simulink model "testemplanner_cs"  (R2023a)
settings: Solver=ode5  StartTime=0.0  StopTime=60  FixedStep=1/1000  RelTol=1e-3
PreLoadFcn:
  | mbxruntime.callbacks.PreLoadFcn(bdroot);
PostLoadFcn:
  | mbxruntime.callbacks.PostLoadFcn(bdroot);
InitFcn:
  | mbxruntime.callbacks.InitFcn(bdroot);
StartFcn:
  | mbxruntime.callbacks.StartFcn(bdroot);
StopFcn:
  | mbxruntime.callbacks.StopFcn(bdroot);
model workspace (MAT data in the model file):
  mbox_table : object (value not decoded)
  model_closed = 0
  sim_status = 0
undefined symbols (not defined in the file): aubr, c_factor, cf, cr, DiscIntNeverNeededParam, global_path_x, global_path_y, KD_PID_distance, KD_PID_speed, KI_PID_distance, KI_PID_speed, KP_PID_distance, KP_PID_speed, la, lb, LQR_K1, LQR_K2, LQR_K3, LQR_K4, m, rack_displacement, right_wheel_ground, tablebr, vubr, vx_break_point
libraries: PreScanSimulinkLibrary x14, Solver_SF x1
(part 7 of 8)

== matlab function testemplanner_cs/Audi_A8_Sedan_1/decision&planning module1/EM Planner/Generate Convex Space&Quadratic Programming/path planning with quadratic programming (qp) ==
  data: qp_path_s output; l_min input; qp_path_l output; l_max input; w_cost_l input; w_cost_dl input; w_cost_ddl input; w_cost_dddl input; w_cost_centre input; w_cost_end_l input; w_cost_end_dl input; w_cost_end_ddl input; host_d1 input; host_d2 input; host_w input; plan_start_s input; plan_start_l input; plan_start_dl input; plan_start_ddl input; qp_path_dl output; qp_path_ddl output; delta_dl_max input; delta_ddl_max input
function [qp_path_s,qp_path_l,qp_path_dl,qp_path_ddl] = ...
fcn(l_min,l_max,w_cost_l,w_cost_dl,w_cost_ddl,w_cost_dddl,w_cost_centre,w_cost_end_l,w_cost_end_dl,w_cost_end_ddl,...
    host_d1,host_d2,host_w,...
    plan_start_s,plan_start_l,plan_start_dl,plan_start_ddl,...
    delta_dl_max,delta_ddl_max)
% 路径二次规划
% 0.5*x'Hx + f'*x = min
% subject to A*x <= b
%            Aeq*x = beq
%            lb <= x <= ub;
% 输入：l_min l_max 点的凸空间
%       w_cost_l 参考线代价
%       w_cost_dl ddl dddl 光滑性代价
%       w_cost_centre 凸空间中央代价
%       w_cost_end_l dl dd1 终点的状态代价 (希望path的终点状态为(0,0,0))
%       host_d1,d2 host质心到前后轴的距离
%       host_w host的宽度
%       plan_start_l,dl,ddl 规划起点
% 输出 qp_path_l dl ddl 二次规划输出的曲线
coder.extrinsic("quadprog");
% 待优化的变量的数量
n = 20;

% 输出初始化
qp_path_l = zeros(n,1);
qp_path_dl = zeros(n,1);
qp_path_ddl = zeros(n,1);
qp_path_s = zeros(n,1);

% H_L H_DL H_DDL H_DDDL Aeq beq A b 初始化
H_L = zeros(3*n, 3*n);
H_DL = zeros(3*n, 3*n);
H_DDL = zeros(3*n, 3*n);
H_DDDL = zeros(n-1, 3*n);
H_CENTRE = zeros(3*n, 3*n);
H_L_END = zeros(3*n, 3*n);
H_DL_END = zeros(3*n, 3*n);
H_DDL_END = zeros(3*n, 3*n);
Aeq = zeros(2*n-2, 3*n);
beq = zeros(2*n-2, 1);
A = zeros(8*n, 3*n);
b = zeros(8*n, 1);
% 更新：加入 dl(i+1) - dl(i) ddl(i+1) - ddl(i) 的约束
A_dl_minus = zeros(n - 1,3*n);
b_dl_minus = zeros(n - 1,1);
A_ddl_minus = zeros(n - 1,3*n);
b_ddl_minus = zeros(n - 1,1);
for i = 1:n-1
    row = i;
    col = 3*i - 2;
    A_dl_minus(row,col:col+5) = [0 -1 0 0 1 0];
    b_dl_minus(row) = delta_dl_max;
    A_ddl_minus(row,col:col+5) = [0 0 -1 0 0 1];
    b_ddl_minus(row) = delta_ddl_max;
end
% -max < a*x < max => ax < max && -ax < -(-max)
A_minus = [A_dl_minus;
          -A_dl_minus;
           A_ddl_minus;
          -A_ddl_minus];
b_minus = [b_dl_minus;
           b_dl_minus;
          b_ddl_minus;
          b_ddl_minus]; 

%  期望的终点状态
end_l_desire = 0;
end_dl_desire = 0;
end_ddl_desire = 0;

% Aeq_sub
ds = 3;%纵向间隔
for i = 1:n
    qp_path_s(i) = plan_start_s + (i-1)*ds;
end

Aeq_sub = [1 ds ds^2/3 -1 0 ds^2/6;
           0 1  ds/2   0 -1 ds/2];
% A_sub;
d1 = host_d1;
d2 = host_d2;
w = host_w;
A_sub = [1  d1 0;
         1  d1 0;
         1 -d2 0;
         1 -d2 0;
        -1 -d1 0;
        -1 -d1 0;
        -1  d2 0;
        -1  d2 0];
% 生成Aeq
for i = 1:n-1
    % 计算分块矩阵左上角的行和列
    row = 2*i - 1;
    col = 3*i - 2;
    Aeq(row:row + 1,col:col + 5) = Aeq_sub;
end
% 生成A
for i = 2:n
    row = 8*i - 7;
    col = 3*i - 2;
    A(row:row + 7,col:col + 2) = A_sub;
end

% 视频里用的找(s(i) - d2,s(i) + d1)的方法过于保守，在这里舍弃掉
% 只要找到四个角点所对应的l_min l_max 即可
% 。。。。。。。。。。。。。。
%    [    .   ]<- 
%    [        ]
% 。。。。。。。。。。。。。
front_index = ceil(d1/ds);
back_index = ceil(d2/ds); % ceil向上取整 ceil(3) = 3 ceil(3.1) = 4
% 生成b
for i = 2:n
    % 左前 右前的index = min(i + front_index,60)
    % 左后 右后的index = max(i - back_index,1)
    % l_min l_max 都是60个点
    index1 = min(3*i - 2 + front_index,n);
    index2 = max(3*i - 2 - back_index,1);
    b(8*i - 7:8*i,1) = [l_max(index1) - w/2;
                        l_max(index1) + w/2;
                        l_max(index2) - w/2;
                        l_max(index2) + w/2;
                       -l_min(index1) + w/2;
                       -l_min(index1) - w/2;
                       -l_min(index2) + w/2;
                       -l_min(index2) - w/2;];
end
%生成 lb ub 主要是对规划起点做约束
lb = ones(3*n,1)*-inf;
ub = ones(3*n,1)*inf;
lb(1) = plan_start_l;
lb(2) = plan_start_dl;
lb(3) = plan_start_ddl;
ub(1) = lb(1);
ub(2) = lb(2);
ub(3) = lb(3);
for i = 2:n
    lb(3*i - 1) = - 2; %约束 l'
    ub(3*i - 1) = 2;
    lb(3*i) = -0.1; %约束 l''
    ub(3*i) = 0.1;
end
% 生成H_L,H_DL,H_DDL,H_CENTRE
for i = 1:n
    H_L(3*i - 2,3*i - 2) = 1;
    H_DL(3*i - 1,3*i - 1) = 1;
    H_DDL(3*i, 3*i) = 1;
end
H_CENTRE = H_L;
% 生成H_DDDL;
H_dddl_sub = [0 0 1 0 0 -1];
for i = 1:n-1
    row = i;
    col = 3*i - 2;
    H_DDDL(row,col:col + 5) = H_dddl_sub;
end
% 生成H_L_END H_DL_END H_DDL_END
H_L_END(3*n - 2,3*n - 2) = 1;
H_DL_END(3*n - 1,3*n - 1) = 1;
H_DDL_END(3*n,3*n) = 1;
% 生成二次规划的H 因为ds ！= 1 所以 dddl = delta_ddl/ds;
H = w_cost_l * (H_L'*H_L) + w_cost_dl * (H_DL'*H_DL) + w_cost_ddl * (H_DDL'*H_DDL)...
   +w_cost_dddl * (H_DDDL'*H_DDDL)/ds + w_cost_centre * (H_CENTRE'*H_CENTRE) + w_cost_end_l * (H_L_END'*H_L_END)...
   +w_cost_end_dl * (H_DL_END'* H_DL_END) + w_cost_ddl * (H_DDL_END'*H_DDL_END);
H = 2 * H;
% 生成f
f = zeros(3*n,1);
 centre_line = 0.5 * (l_min + l_max); % 此时centre line 还是60个点
% centre_line = dp_path_l_final;
for i = 1:n
    f(3*i - 2) = -2 * centre_line(3*i - 2);
end
% 避免centreline权重过大影响轨迹平顺性
for i = 1:n
    if abs(f(i)) > 0.3
        f(i) = w_cost_centre * f(i);
    end
end
% 终点要接近end_l dl ddl desire
f(3*n - 2) = f(3*n - 2) -2 * end_l_desire * w_cost_end_l;
f(3*n - 1) = f(3*n - 1) -2 * end_dl_desire * w_cost_end_dl;
f(3*n) = f(3*n) -2 * end_ddl_desire * w_cost_end_ddl;

% f = f*H_L';

X = quadprog(H,f,[A;A_minus],[b;b_minus],Aeq,beq,lb,ub);

for i = 1:n
    qp_path_l(i) = X(3*i - 2);
    qp_path_dl(i) = X(3*i - 1);
    qp_path_ddl(i) = X(3*i);
end

end

== matlab function testemplanner_cs/Audi_A8_Sedan_1/decision&planning module1/EM Planner/Obs/Cartesian2Frenet-static obs/S&L calcu ==
  data: s_set output; l_set output; x_set input; y_set input; proj_x_set input; proj_y_set input; proj_heading_set input; index2s input; planning_start_match_point_index input; frenet_x input; frenet_y input
function [s_set, l_set] = fcn(x_set, y_set, proj_x_set, proj_y_set, proj_heading_set, index2s, ...
    planning_start_match_point_index, frenet_x, frenet_y)

%此函数用来存储规划起点及障碍物在以自车定位的投影点为参考线原点的frenet坐标系的sl坐标
%由于不知道规划起点及障碍物共多少个，故需要缓冲
%计算s时直接复用index2s模块中写好的子函数
%共有128个点

n = 128;
s_set = ones(n,1)*nan;
l_set = ones(n,1)*nan;
 
for i = 1:length(x_set)
    if isnan(x_set(i))
        break;
    end
    %计算规划起点或障碍物的匹配点到参考线原点(自车在参考线上的投影点)的弧长
    s_set(i) = CalcSFromIndex2s(index2s, planning_start_match_point_index(i), proj_x_set(i), proj_y_set(i), frenet_x, frenet_y);
    vector_rh = [x_set(i); y_set(i)];
    vector_rr = [proj_x_set(i); proj_y_set(i)];
    vector_nor_r = [-sin(proj_heading_set(i)); cos(proj_heading_set(i))];
    l_set(i) = (vector_rh-vector_rr)'*vector_nor_r;
end
end

%复用index2s中写好的计算弧长s的子函数
function s0 = CalcSFromIndex2s(index2s, match_point_index, proj_x, proj_y, path_x, path_y)
%该函数第一次调用时用来计算自车投影点到参考线起点的弧长！！！
%该函数复用时用来计算障碍物投影点到参考线原点的弧长！！！
%我认为这里第一次使用与复用时的逻辑混乱，非常复杂

%我们要计算参考线起点到投影点（坐标系原点）的弧长
%并且已知参考线起点到匹配点的弧长index2s（i）
%所以要计算投影点与匹配点间的距离和相对位置关系
%向量的内积可以判断位置关系

%先定义投影点与匹配点的误差向量
vector1 = [proj_x; proj_y]-[path_x(match_point_index); path_y(match_point_index)];

%可以根据匹配点的临近点近似描述匹配点的方向向量
%1：如果匹配点前面还有点
%2：如果匹配点是最后一个点
if match_point_index < length(path_x)
    %定义匹配点的切向量
    vector2 = [path_x(match_point_index+1)-path_x(match_point_index); path_y(match_point_index+1)-path_y(match_point_index)];
else
    vector2 = [path_x(match_point_index)-path_x(match_point_index-1); path_y(match_point_index)-path_y(match_point_index-1)];
end

%判断匹配点与投影点的相对位置关系
%计算参考线起点到投影点的弧长
if vector1'*vector2 > 0
    %投影点在前，匹配点在后
    s0 = index2s(match_point_index)+sqrt(vector1'*vector1);
else
    %匹配点在前，投影点在后
    s0 = index2s(match_point_index)-sqrt(vector1'*vector1);
end
end

== matlab function testemplanner_cs/Audi_A8_Sedan_1/decision&planning module1/EM Planner/Obs/Cartesian2Frenet-static obs/S_dot&L_dot&dL calcu  ==
  data: s_dot_set output; vx_set input; vy_set input; proj_heading_set input; proj_kappa_set input; l_set input; l_dot_set output; dl_set output
function [s_dot_set, l_dot_set, dl_set]  = fcn(vx_set, vy_set, proj_heading_set, proj_kappa_set, l_set)

%这个函数用来存储s_dot&l_dot&dl的集合
n = 128;
s_dot_set = ones(n,1)*nan;
l_dot_set = ones(n,1)*nan;
dl_set = ones(n,1)*nan;

for i = 1:length(l_set)
    if isnan(l_set(i))
        break;
    end
    vector_vh = [vx_set(i); vy_set(i)];
    vector_tor_r = [cos(proj_heading_set(i)); sin(proj_heading_set(i))];
    vector_nor_r = [-sin(proj_heading_set(i)); cos(proj_heading_set(i))];
    s_dot_set(i) = vector_vh'*vector_tor_r/(1-proj_kappa_set(i)*l_set(i));
    l_dot_set(i) = vector_vh'*vector_nor_r;

    %dl=l_dot/s_dot,所以s_dot不能为0，这里要打一个补丁，当s_dot趋于0时，dl=0
    if abs(s_dot_set(i)) < 1e-6
        dl_set(i) = 0;
    else
        dl_set(i) = l_dot_set(i)/s_dot_set(i);
    end

end

end

== matlab function testemplanner_cs/Audi_A8_Sedan_1/control module/control main/chassic steering system/MATLAB Function ==
  data: u input; right_steer output; la input; lb input
function right_steer = fcn(u,la,lb)
if abs(u)<1e-2
   right_steer = u;
else
   R =  (la+lb)/tan(u);
   right_steer = atan((la+lb)/(R+1.624/2));
end

== matlab function testemplanner_cs/Audi_A8_Sedan_1/decision&planning module1/EM Planner/Obs/Cartesian2Frenet-static obs/S_dot2&L_dot2&ddL calcu ==
  data: ax_set input; s_dot2_set output; ay_set input; proj_heading_set input; proj_kappa_set input; l_set input; dl_set input; s_dot_set input; l_dot2_set output; ddl_set output
function [s_dot2_set, l_dot2_set, ddl_set] = fcn(ax_set, ay_set, proj_heading_set, proj_kappa_set, l_set, dl_set...
    , s_dot_set)

%该函数用来存储s_dot2&l_dot2&ddl,同样要设置缓冲
n = 128;
s_dot2_set = ones(n,1)*nan;
l_dot2_set = ones(n,1)*nan; 
ddl_set = ones(n,1)*nan;

for i = 1:length(l_set)
    if isnan(l_set(i))
        break;
    end
    vector_ah = [ax_set(i); ay_set(i)];
    vector_tor_r = [cos(proj_heading_set(i)); sin(proj_heading_set(i))];
    vector_nor_r = [-sin(proj_heading_set(i)); cos(proj_heading_set(i))];

    %kr'=dkr/ds,曲率随弧长的变化速率很小，kr'=0
    s_dot2_set(i) = vector_ah'*vector_tor_r/(1-proj_kappa_set(i)*l_set(i))+proj_kappa_set(i)*dl_set(i)*s_dot_set(i)^2/(1-proj_kappa_set(i)*l_set(i))...
        +s_dot_set(i)^2*proj_kappa_set(i)*dl_set(i)/(1-proj_kappa_set(i)*l_set(i));

    l_dot2_set(i) = vector_ah'*vector_nor_r-proj_kappa_set(i)*s_dot_set(i)^2*(1-proj_kappa_set(i)*l_set(i));

    %ddl的表达式分母上有s_dot,同样要确保s_dot不为0
    if abs(s_dot_set(i)) < 1e-6
        ddl_set(i) = 0;
    else
        ddl_set(i) = (l_dot2_set(i)-dl_set(i)*s_dot2_set(i))/s_dot_set(i)^2; 
    end

end

end

== matlab function testemplanner_cs/Audi_A8_Sedan_1/decision&planning module1/EM Planner/Obs/Obs Filter ==
  data: host_x input; obs_x_final_set output; host_y input; obs_x_set_gcs input; obs_y_set_gcs input; obs_velocity_set_gcs input; obs_heading_set_gcs input; host_heading_xy input; obs_y_final_set output; obs_velocity_final_set output; obs_heading_final_set output
function [obs_x_final_set, obs_y_final_set, obs_velocity_final_set, obs_heading_final_set] = fcn(host_x, host_y, obs_x_set_gcs, ...
    obs_y_set_gcs, obs_velocity_set_gcs, obs_heading_set_gcs, host_heading_xy)

%该函数用来筛选范围内的障碍物（包括静态和动态）
%筛选纵向-10：60，横向-10：10范围内单车道上的障碍物
%完全体的EMPLANNER是多车道并行计算
%传感器最多识别32个障碍物，需要设置缓冲

n = 32;
obs_x_final_set = ones(n,1)*nan;
obs_y_final_set = ones(n,1)*nan;
obs_velocity_final_set = ones(n,1)*nan;
obs_heading_final_set = ones(n,1)*nan;
count = 1;

%通过障碍物与自车间的距离判断
for i = 1:length(obs_x_set_gcs)
    if isnan(obs_x_set_gcs(i))
        break;
    end
    vector_err = [obs_x_set_gcs(i); obs_y_set_gcs(i)]-[host_x; host_y];
    vector_tor_h = [cos(host_heading_xy); sin(host_heading_xy)];
    vector_nor_h = [-sin(host_heading_xy); cos(host_heading_xy)];
    %车身坐标系下的纵向距离及横向距离
    distant_long = vector_err'*vector_tor_h;
    distant_later = vector_err'*vector_nor_h;

    if distant_long < 60 && distant_long > -10 && distant_later > -10 && distant_later < 10
        obs_x_final_set(count) = obs_x_set_gcs(i);
        obs_y_final_set(count) = obs_y_set_gcs(i);
        obs_velocity_final_set(count) = obs_velocity_set_gcs(i);
        obs_heading_final_set(count) = obs_heading_set_gcs(i);
        count = count+1;
    end
end



end

== matlab function testemplanner_cs/Audi_A8_Sedan_1/decision&planning module1/EM Planner/Obs/Static&Dynamic Obs Filter ==
  data: obs_x_final_set input; static_obs_x_set output; obs_y_final_set input; obs_velocity_final_set input; obs_heading_final_set input; static_obs_y_set output; dynamic_obs_x_set output; dynamic_obs_y_set output; dynamic_obs_vx_set output; dynamic_obs_vy_set output
function [static_obs_x_set, static_obs_y_set, ...
    dynamic_obs_x_set, dynamic_obs_y_set, dynamic_obs_vx_set, dynamic_obs_vy_set] = fcn(...
    obs_x_final_set, obs_y_final_set, obs_velocity_final_set, obs_heading_final_set)

%该函数的作用是把范围内的静/动态障碍物分离开来
%根据障碍物速度的大小作为判断障碍物静动态的准则
%还是要做缓冲

n = 32;
static_obs_x_set = ones(n,1)*nan;
static_obs_y_set = ones(n,1)*nan;
% static_obs_velocity_set = ones(n,1)*nan;
% static_obs_heading_set = ones(n,1)*nan;
dynamic_obs_x_set = ones(n,1)*nan;
dynamic_obs_y_set = ones(n,1)*nan;
dynamic_obs_vx_set = ones(n,1)*nan;
dynamic_obs_vy_set = ones(n,1)*nan;
static_count = 1;
dynamic_count = 1;

for i = 1:length(obs_x_final_set)
    if isnan(obs_x_final_set(i))
        break;
    end
    if abs(obs_velocity_final_set(i)) < 0.1
        %属于静态障碍物
        static_obs_x_set(static_count) = obs_x_final_set(i);
        static_obs_y_set(static_count) = obs_y_final_set(i);
        % static_obs_velocity_set(static_count) = obs_velocity_final_set(i);
        % static_obs_heading_set(static_count) = obs_heading_final_set(i);
        static_count = static_count+1;
    else
        %属于动态障碍物
        dynamic_obs_x_set(dynamic_count) = obs_x_final_set(i);
        dynamic_obs_y_set(dynamic_count) = obs_y_final_set(i);
        % dynamic_obs_velocity_set(dynamic_count) = obs_velocity_final_set(i);
        % dynamic_obs_heading_set(dynamic_count) = obs_heading_final_set(i);
        dynamic_count = dynamic_count+1;
    end
end





end

== matlab function testemplanner_cs/Audi_A8_Sedan_1/decision&planning module1/EM Planner/Obs/match&proj point search2 ==
  data: match_point_index_set output; proj_x_set output; proj_y_set output; proj_heading_set output; proj_kappa_set output; x_set input; y_set input; frenet_x_set input; frenet_y_set input; frenet_heading_set input; frenet_kapppa_set input
function [match_point_index_set, proj_x_set, proj_y_set, proj_heading_set, proj_kappa_set] = fcn(x_set, y_set, frenet_x_set, frenet_y_set, ...
    frenet_heading_set, frenet_kapppa_set)

%待投影点是一个集合（自车，障碍物），每一个点分别遍历寻找匹配点，再寻找投影点
%匹配点集合要保存下来，作为下次遍历开始的起点
%第一次遍历，没有任何提示，从frenet点集第一点开始遍历
%若不是第一次遍历，从上次保存的匹配点开始，注意方向
%待投影点-寻找匹配点-寻找投影点-投影点（x,y,heading,kappa），保存匹配点索引集合

%（待）投影点数量未知，设置缓冲，最多批量处理128个点,信息冗余用NAN（not a number）处理
n = 128;
match_point_index_set = ones(n,1)*nan;
proj_x_set = ones(n,1)*nan;
proj_y_set = ones(n,1)*nan;
proj_heading_set = ones(n,1)*nan;
proj_kappa_set = ones(n,1)*nan;

%两种情况：第一次遍历，非第一次遍历
%声明两个全局变量，第一个用来判断是否初次运行，第二个用来存储上次匹配点集合
persistent is_first_run
persistent pre_match_point_index_set
persistent pre_x_set
persistent pre_y_set
persistent pre_frenet_x_set;
persistent pre_frenet_y_set;
persistent pre_frenet_heading_set;

if isempty(is_first_run)
    is_first_run = 0;
    pre_match_point_index_set = ones(n,1)*nan;
    %遍历每一个点寻找匹配点
    start_search_index = 1;
    for i = 1:length(x_set)
        if isnan(x_set(i))
            break;
        end
        increase_count = 0;
        min_distant = inf;
        for j = start_search_index:length(frenet_x_set)
            distant = (x_set(i)-frenet_x_set(j))^2+(y_set(i)-frenet_y_set(j))^2;
            if distant < min_distant
                min_distant = distant;
                increase_count = 0;
                match_point_index_set(i) = j;
            else
                increase_count = increase_count+1;
            end
            %第一次遍历连续增加50次停止
            if increase_count > 50
                break;
            end
        end
        %通过匹配点计算投影点
        %计算匹配点的位矢及方向向量
        vector_match_point = [frenet_x_set(match_point_index_set(i));frenet_y_set(match_point_index_set(i))];
        vector_match_point_direction = [cos(frenet_heading_set(match_point_index_set(i)));sin(frenet_heading_set(match_point_index_set(i)))];
        vector_d = [x_set(i);y_set(i)]-vector_match_point;
        ds = vector_d'*vector_match_point_direction;
        vector_ds = ds*vector_match_point_direction;
        vector_proj_point = vector_match_point+vector_ds;
        %计算投影点的x,y,heading,kappa
        proj_x_set(i) = vector_proj_point(1);
        proj_y_set(i) = vector_proj_point(2);
        proj_heading_set(i) = frenet_heading_set(match_point_index_set(i))+frenet_kapppa_set(match_point_index_set(i))*ds;
        proj_kappa_set(i) = frenet_kapppa_set(match_point_index_set(i));
    end
    pre_match_point_index_set = match_point_index_set;
    pre_frenet_x_set = frenet_x_set;
    pre_frenet_y_set = frenet_y_set;
    pre_frenet_heading_set = frenet_heading_set;
    pre_x_set = x_set;
    pre_y_set = y_set;
else
    %如果不是第一次遍历
    for i = 1:length(x_set)

        if isnan(x_set(i))
            break;
        end
        %下面这行代码有严重问题，需要投影的不仅是自车，还有障碍物
        %而第一次运行时传感器可能监测不到障碍物，即算法会跳过is first run分支执行else分支
        %此时pre_match_point_index_set中除了自车都是nan，所以需要修复
        start_search_index = pre_match_point_index_set(i);
        increase_count_limit = 5;

        %下面是修复一个bug，pre_match_point_index(i)与x_set(i)不一定是同一个障碍物
        square_dis = (x_set(i)-pre_x_set(i))^2+(y_set(i)-pre_y_set(i))^2;
        if square_dis > 36
            start_search_index = nan;
        end

        if isnan(start_search_index)
            %从第一个点开始遍历，并需要遍历50次防止取到局部极小值
            increase_count_limit = 50;
            start_search_index = 1;
        end

        increase_count = 0;
        min_distant = inf;
        %判断遍历方向
        vector_pre_match_point = [pre_frenet_x_set(start_search_index);pre_frenet_y_set(start_search_index)];
        vector_pre_match_point_direction = [cos(pre_frenet_heading_set(start_search_index));sin(pre_frenet_heading_set(start_search_index))];
        flag = ([x_set(i);y_set(i)]-vector_pre_match_point)'*vector_pre_match_point_direction;
        

        %正向遍历
        if flag > 0.001
            for j = start_search_index:length(frenet_x_set)
                distant = (x_set(i)-frenet_x_set(j))^2+(y_set(i)-frenet_y_set(j))^2;
                if distant < min_distant
                    min_distant = distant;
                    increase_count = 0;
                    match_point_index_set(i) = j;
                else
                    increase_count = increase_count+1;
                end
                %连续增加5次停止
                if increase_count > increase_count_limit
                    break;
                end
            end
            % %通过匹配点计算投影点
            % %计算匹配点的位矢及方向向量
            % vector_match_point = [frenet_x_set(match_point_index_set(i));frenet_y_set(match_point_index_set(i))];
            % vector_match_point_direction = [cos(frenet_heading_set(match_point_index_set(i)));sin(frenet_heading_set(match_point_index_set(i)))];
            % vector_d = [x_set(i);y_set(i)]-vector_match_point;
            % ds = vector_d'*vector_match_point_direction;
            % vector_ds = ds*vector_match_point_direction;
            % vector_proj_point = vector_match_point+vector_ds;
            % %计算投影点的x,y,heading,kappa
            % proj_x_set(i) = vector_proj_point(1);
            % proj_y_set(i) = vector_proj_point(2);
            % proj_heading_set(i) = frenet_heading_set(match_point_index_set(i))+frenet_kapppa_set(match_point_index_set(i))*ds;
            % proj_kappa_set(i) = frenet_kapppa_set(match_point_index_set(i));
        elseif flag < -0.001
            %反向遍历
             for j = start_search_index:-1:1
                distant = (x_set(i)-frenet_x_set(j))^2+(y_set(i)-frenet_y_set(j))^2;
                if distant < min_distant
                    min_distant = distant;
                    increase_count = 0;
                    match_point_index_set(i) = j;
                else
                    increase_count = increase_count+1;
                end
                %连续增加5次停止
                if increase_count > increase_count_limit
                    break;
                end
            end
        else
            match_point_index_set(i) = start_search_index;
        end

        %通过匹配点计算投影点
        %计算匹配点的位矢及方向向量
        vector_match_point = [frenet_x_set(match_point_index_set(i));frenet_y_set(match_point_index_set(i))];
        vector_match_point_direction = [cos(frenet_heading_set(match_point_index_set(i)));sin(frenet_heading_set(match_point_index_set(i)))];
        vector_d = [x_set(i);y_set(i)]-vector_match_point;
        ds = vector_d'*vector_match_point_direction;
        vector_ds = ds*vector_match_point_direction;
        vector_proj_point = vector_match_point+vector_ds;
        %计算投影点的x,y,heading,kappa
        proj_x_set(i) = vector_proj_point(1);
        proj_y_set(i) = vector_proj_point(2);
        proj_heading_set(i) = frenet_heading_set(match_point_index_set(i))+frenet_kapppa_set(match_point_index_set(i))*ds;
        proj_kappa_set(i) = frenet_kapppa_set(match_point_index_set(i));

    end
    pre_match_point_index_set = match_point_index_set;
    pre_frenet_x_set = frenet_x_set;
    pre_frenet_y_set = frenet_y_set;
    pre_frenet_heading_set = frenet_heading_set;
    pre_x_set = x_set;
    pre_y_set = y_set;
end

== matlab function testemplanner_cs/Audi_A8_Sedan_1/decision&planning module1/EM Planner/cacul planning start gcs ==
  data: pre_trajectory_x input; planning_start_x output; pre_trajectory_y input; pre_trajectory_heading input; pre_trajectory_kappa input; pre_trajectory_speed input; pre_trajectory_accel input; pre_trajectory_time input; current_time input; host_x input; host_y input; host_heading_xy input; host_vx input; host_vy input; host_ax input; host_ay input; planning_start_y output; planning_start_heading output; planning_start_kappa output; planning_start_vx output; planning_start_vy output; planning_start_ax output; planning_start_ay output; planning_start_time output; stitch_x output; stitch_y output; stitch_heading output; stitch_kappa output; stitch_speed output; stitch_accel output; stitch_time output
function [planning_start_x, planning_start_y, planning_start_heading, planning_start_kappa, planning_start_vx, ...
    planning_start_vy, planning_start_ax, planning_start_ay, planning_start_time, stitch_x, stitch_y, stitch_heading, stitch_kappa, ...
    stitch_speed, stitch_accel, stitch_time] = fcn(pre_trajectory_x, pre_trajectory_y, pre_trajectory_heading, ...
    pre_trajectory_kappa, pre_trajectory_speed,  pre_trajectory_accel, pre_trajectory_time, current_time, host_x, ...
    host_y, host_heading_xy, host_vx, host_vy, host_ax, host_ay)


%该模块用来计算规划起点的信息：x,y,heading,kappa,vx,vy,ax,ay
%以及待拼接的轨迹信息：stitch_x,y,heading,kappa...
%输入参数：hostx,y,heading,kappa是世界坐标系下，而vx,vy,ax,ay是基于车辆坐标系
%输出参数：规划开始点以及待拼接轨迹的vx,vy,ax,ay都是基于世界坐标系
%stitch用来存储规划起点前20个点的轨迹，要生成缓冲矩阵

stitch_x = zeros(20,1);
stitch_y = zeros(20,1);
stitch_heading = zeros(20,1);
stitch_kappa = zeros(20,1);
stitch_speed = zeros(20,1);
stitch_accel = zeros(20,1);
%待拼接矩阵的时间序列，用-1代表无需拼接
stitch_time = ones(20,1)*-1;

%定义持久变量，若是第一次运行...
%若不是第一次运行...
persistent is_first_run
if isempty(is_first_run)
    is_first_run = 0;
    %第一次运行时没有上一周期的规划结果，可以根据车辆运动学模型递推出current_time+100ms时的状态
    %但第一次运行时，没有初始车速、加速度，也不需要轨迹拼接，直接拿定位信息当作规划起点即可
    planning_start_x = host_x; 
    planning_start_y = host_y;
    planning_start_heading = host_heading_xy;
    planning_start_kappa = 0;
    %下面这一行是老王的写法，有疑问
    % planning_start_kappa = 0;
    planning_start_vx = 0;
    planning_start_vy = 0;
    planning_start_ax = 0;
    planning_start_ay = 0;
    %planning_start_time为规划起点对应的时间戳，而不是规划开始的时间
    planning_start_time = current_time+0.1;

else
    %若不是第一次运行
    %首先要在上周期规划的轨迹中寻找current所对应的索引的信息（应该处在什么位置），根据实际所处位置做出判断控制的效果、是否需要拼接轨迹及规划起点
    for i = 1:length(pre_trajectory_time)-1
        if pre_trajectory_time(i) <= current_time && pre_trajectory_time(i+1) > current_time
            break;
        end
    end
    %遍历出的i即为current_time所对应的序号
    %根据定位位置与理想位置之间的误差判断是否需要轨迹拼接
    x_current = host_x;
    y_current = host_y;   
    heading_current = host_heading_xy;
    %kappa_current = 0; %老王的写法，为什么现在的曲率是0？
    kappa_current = 0;
    %定位的vxvy...是基于车辆坐标系的，要转换成世界坐标系
    vx_current = host_vx*cos(heading_current)-host_vy*sin(heading_current);
    vy_current = host_vy*cos(heading_current)+host_vx*sin(heading_current);
    ax_current = host_ax*cos(heading_current)-host_ay*sin(heading_current);
    ay_current = host_ay*cos(heading_current)+host_ax*sin(heading_current);
    x_desire = pre_trajectory_x(i);
    y_desire = pre_trajectory_y(i);
    heading_desire = pre_trajectory_heading(i);
    tor1 = [cos(heading_desire); sin(heading_desire)];
    nor1 = [-sin(heading_desire); cos(heading_desire)];
    %根据误差向量及切向量和法向量计算定位和理想位置间的横向误差及纵向误差
    err_vector = [x_current; y_current]-[x_desire; y_desire];
    %纵向误差
    err_long = abs(err_vector'*tor1);
    %侧向误差
    err_lat = abs(err_vector'*nor1);
    %规划的周期是100ms，即0.1s
    dt = 0.1;
    %判断控制是否跟上了轨迹,一般认为纵向误差大于2或者横向误差大于0.5时控制效果差
    if err_long > 2.5 || err_lat > 0.5
        %控制没有跟上轨迹，需要根据车辆运动学模型递推一个周期得到规划起点的状态,这里认为车辆在一个周期内做匀加速直线运动
        planning_start_x = x_current+vx_current*dt+0.5*ax_current*dt^2;
        planning_start_y = y_current+vy_current*dt+0.5*ay_current*dt^2;
        
        planning_start_kappa = kappa_current;
        planning_start_vx = vx_current+ax_current*dt;
        planning_start_vy = vy_current+ay_current*dt;
        planning_start_heading = atan2(planning_start_vy,planning_start_vx);
        planning_start_ax = ax_current;
        planning_start_ay = ay_current;
        %把planning_start_time（规划开始时间）表述为current_time+0.1是否不妥，规划开始时间应为current_time,此处仍有疑问
        planning_start_time = current_time+0.1;
        %控制没有跟上规划，递推出下个周期规划起点后再拿上周期的规划结果做轨迹拼接也就没有意义
    else
        %控制跟上了规划，需要做轨迹拼接
        %规划起点是current_time+0.1在时间戳里对应的索引对应的信息
        %先找到规划起点的索引
        for j = i:length(pre_trajectory_time)-1
            if pre_trajectory_time(j) <= current_time+0.1 && pre_trajectory_time(j+1) > current_time+0.1
                break;
            end
        end
        %j即为current_time+0.1在pre_trajectory_time时间戳里的索引
        planning_start_x = pre_trajectory_x(j);
        planning_start_y = pre_trajectory_y(j);
        %pre_trajecctory_speed,accel为轨迹的切向速度、加速度
        planning_start_heading = pre_trajectory_heading(j);
        planning_start_kappa = pre_trajectory_kappa(j);
        planning_start_vx = pre_trajectory_speed(j)*cos(planning_start_heading);
        planning_start_vy = pre_trajectory_speed(j)*sin(planning_start_heading);
        %加速度分为切向加速度和法向加速度
        %计算规划起点的切向量和法向量
        tor2 = [cos(planning_start_heading); sin(planning_start_heading)];
        nor2 = [-sin(planning_start_heading); cos(planning_start_heading)];
        %计算规划起点的切向加速度和法向加速度
        a_tor = pre_trajectory_accel(j)*tor2;
        a_nor = pre_trajectory_speed(j)^2*planning_start_kappa*nor2;
        planning_start_ax = a_tor(1)+a_nor(1);
        planning_start_ay = a_tor(2)+a_nor(2);
        %下面的规划开始时间同样有疑问
        % planning_start_time = pre_trajectory_time(j);  
        planning_start_time = current_time+0.1;

        %下面开始准备轨迹拼接，分为规划起点之前足够20个点和不足20个点两种情况
        if j > 20
            stitch_x = pre_trajectory_x(j-20:j-1);
            stitch_y = pre_trajectory_y(j-20:j-1);
            stitch_heading = pre_trajectory_heading(j-20:j-1);
            stitch_kappa = pre_trajectory_kappa(j-20:j-1);
            stitch_speed = pre_trajectory_speed(j-20:j-1);
            stitch_accel = pre_trajectory_accel(j-20:j-1);
            stitch_time = pre_trajectory_time(j-20:j-1);
        else
            %q:如果j=1怎么办？
            %a：只要i！=j，j就不会为1；即current_time的索引不能等于current_time+0.1的索引
            %轨迹点的采样要足够密集；eg:如果1s采样一个点，则会i=j...
            stitch_x(22-j:20) = pre_trajectory_x(1:j-1);
            stitch_y(22-j:20) = pre_trajectory_y(1:j-1);
            stitch_heading(22-j:20) = pre_trajectory_heading(1:j-1);
            stitch_kappa(22-j:20) = pre_trajectory_kappa(1:j-1);
            stitch_speed(22-j:20) = pre_trajectory_speed(1:j-1);
            stitch_accel(22-j:20) = pre_trajectory_accel(1:j-1);
            stitch_time(22-j:20) = pre_trajectory_time(1:j-1);
        end
    end

end

== stateflow chart testemplanner_cs/Audi_A8_Sedan_1/Chart ==
  (default) -> (junction 5)
  (junction 5) -> (junction 7)
  (junction 7) -> (junction 9) [order 1] : [i >= 100]
  (junction 7) -> (junction 13) [order 2] : {
      | i = i+1;
      | }
  (junction 9) -> (junction 11) : {
      | do_planning;
      | i = 1;
      | }
  (junction 11) -> (junction 13)
  (junction 13) -> (junction 16)
  (junction 16) -> (junction 18) [order 1] : [j >= 10]
  (junction 16) -> (junction 22) [order 2] : {
      | j = j+1;
      | }
  (junction 18) -> (junction 20) : {
      | do_control;
      | j = 1;
      | }
  (junction 20) -> (junction 22)
  (junction 22) -> (junction 25)
  data: i local =1; j local =1
  events: do_planning output FUNCTION_CALL_EVENT; do_control output FUNCTION_CALL_EVENT

== matlab function testemplanner_cs/Audi_A8_Sedan_1/decision&planning module1/EM Planner/calc path length and map between point and s ==
  data: trajectory_x input; path_s_end output; trajectory_y input; path_s output
function [path_s_end,path_s] = fcn(trajectory_x,trajectory_y)
% 该函数将计算以trajectory的s 与 x y 的对应关系，可以看作是trajectory index2s
n = length(trajectory_x);
path_s = zeros(n,1);
sum = 0;
for i = 2:length(trajectory_x)
    if isnan(trajectory_x(i))
        break;
    end
    sum = sum + sqrt((trajectory_x(i) - trajectory_x(i-1))^2 + (trajectory_y(i) - trajectory_y(i-1))^2);
    path_s(i) = sum;
end
% 计算出trajectory的长度
if i == n
    path_s_end = path_s(end);
else
    % 因为循环的退出条件为isnan(trajectory_x(i)) 所以 i 所对应的数为 nan 
    path_s_end = path_s(i - 1);
end

== matlab function testemplanner_cs/Audi_A8_Sedan_1/decision&planning module1/EM Planner/calc speed planning start condition ==
  data: plan_start_vx input; plan_start_s_dot output; plan_start_vy input; plan_start_ax input; plan_start_ay input; plan_start_heading input; plan_start_s_dot2 output
function [plan_start_s_dot,plan_start_s_dot2] = fcn(plan_start_vx,plan_start_vy,plan_start_ax,plan_start_ay,plan_start_heading)
% 该函数计算速度规划的初始条件
tor = [cos(plan_start_heading);sin(plan_start_heading)];
v_t = tor'*[plan_start_vx;plan_start_vy];
a_t = tor'*[plan_start_ax;plan_start_ay];
plan_start_s_dot = v_t;
plan_start_s_dot2 = a_t;

== matlab function testemplanner_cs/Audi_A8_Sedan_1/decision&planning module1/EM Planner/generate index2s ==
  data: origin_match_point_index input; index2s output; origin_proj_x input; origin_proj_y input; path_x input; path_y input
function index2s = fcn(origin_match_point_index, origin_proj_x, origin_proj_y, path_x, path_y)

%该函数用来计算索引序号i对应的弧长s,对于每一个待投影的物体，都有一个匹配点（索引），index2s即为参考线原点到匹配点的弧长
%先计算索引点到参考线起始点的弧长
%再计算参考线起始点到自然坐标系原点（自车投影点）的弧长，作差得到frenet坐标系原点到索引点的弧长
%因为参考线有181个点，对应181个弧长(有一个点是坐标原点，该点到原点的距离认为是0)
n = 181;
index2s = zeros(n,1);
index2s(1) = 0;
for i = 2:n
    index2s(i) = sqrt((path_x(i)-path_x(i-1))^2+(path_y(i)-path_y(i-1))^2)+index2s(i-1);
end

%s0是一个通用函数，用来计算投影点到参考线原点的弧长(第一次调用时计算投影点到参考线起点的弧长)
s0 = CalcSFromIndex2s(index2s, origin_match_point_index, origin_proj_x, origin_proj_y, path_x, path_y);
index2s = index2s-ones(n,1)*s0;

end

%定义上述通用函数
function s0 = CalcSFromIndex2s(index2s, match_point_index, proj_x, proj_y, path_x, path_y)
%该函数第一次调用时用来计算自车投影点到参考线起点的弧长！！！
%该函数复用时用来计算障碍物投影点到参考线原点的弧长！！！
%我认为这里第一次使用与复用时的逻辑混乱，非常复杂

%我们要计算参考线起点到投影点（坐标系原点）的弧长
%并且已知参考线起点到匹配点的弧长index2s（i）
%所以要计算投影点与匹配点间的距离和相对位置关系
%向量的内积可以判断位置关系

%先定义投影点与匹配点的误差向量
vector1 = [proj_x; proj_y]-[path_x(match_point_index); path_y(match_point_index)];

%可以根据匹配点的临近点近似描述匹配点的方向向量
%1：如果匹配点前面还有点
%2：如果匹配点是最后一个点
if match_point_index < length(path_x)
    %定义匹配点的切向量
    vector2 = [path_x(match_point_index+1)-path_x(match_point_index); path_y(match_point_index+1)-path_y(match_point_index)];
else
    vector2 = [path_x(match_point_index)-path_x(match_point_index-1); path_y(match_point_index)-path_y(match_point_index-1)];
end

%判断匹配点与投影点的相对位置关系
%计算参考线起点到投影点的弧长
if vector1'*vector2 > 0
    %投影点在前，匹配点在后
    s0 = index2s(match_point_index)+sqrt(vector1'*vector1);
else
    %匹配点在前，投影点在后
    s0 = index2s(match_point_index)-sqrt(vector1'*vector1);
end
end

== matlab function testemplanner_cs/Audi_A8_Sedan_1/decision&planning module1/EM Planner/increase st point count ==
  data: s_init input; s output; s_dot_init input; s_dot2_init input; relative_time_init input; s_dot output; s_dot2 output; relative_time output
function [s,s_dot,s_dot2,relative_time] = fcn(s_init,s_dot_init,s_dot2_init,relative_time_init)
%该函数将增密s s_dot s_dot2
% 为什么需要增密，因为控制的执行频率是规划的10倍，轨迹点如果不够密，必然会导致规划效果不好
% 但是若在速度二次规划中点取的太多，会导致二次规划的矩阵规模太大计算太慢
% 所以方法是在二次规划中选取少量的点优化完毕后，在用此函数增密
T = relative_time_init(end);
n = 401;
dt = T/(n-1);
s = zeros(n,1);
s_dot = zeros(n,1);
s_dot2 = zeros(n,1);
relative_time = zeros(n,1);
for i = 1:n
    current_t = (i-1)*dt;
    for j = 1:length(relative_time_init)-1
        if relative_time_init(j) <= current_t && relative_time_init(j+1) > current_t
            break;
        end
    end
    x = current_t - relative_time_init(j);
    s(i) = s_init(j) + s_dot_init(j)*x + (1/3)*s_dot2_init(j)*x^2 + (1/6)*s_dot2_init(j+1)*x^2; 
    s_dot(i) = s_dot_init(j) + 0.5*s_dot2_init(j)*x + 0.5*s_dot2_init(j+1)*x;
    s_dot2(i) = s_dot2_init(j) + (s_dot2_init(j+1) - s_dot2_init(j))*x/(relative_time_init(j+1) - relative_time_init(j));
    relative_time(i) = current_t;
end

== matlab function testemplanner_cs/Audi_A8_Sedan_1/decision&planning module1/EM Planner/match&proj point search2 ==
  data: match_point_index_set output; proj_x_set output; proj_y_set output; proj_heading_set output; proj_kappa_set output; x_set input; y_set input; frenet_x_set input; frenet_y_set input; frenet_heading_set input; frenet_kapppa_set input
function [match_point_index_set, proj_x_set, proj_y_set, proj_heading_set, proj_kappa_set] = fcn(x_set, y_set, frenet_x_set, frenet_y_set, ...
    frenet_heading_set, frenet_kapppa_set)

%待投影点是一个集合（自车，障碍物），每一个点分别遍历寻找匹配点，再寻找投影点
%匹配点集合要保存下来，作为下次遍历开始的起点
%第一次遍历，没有任何提示，从frenet点集第一点开始遍历
%若不是第一次遍历，从上次保存的匹配点开始，注意方向
%待投影点-寻找匹配点-寻找投影点-投影点（x,y,heading,kappa），保存匹配点索引集合

%（待）投影点数量未知，设置缓冲，最多批量处理128个点,信息冗余用NAN（not a number）处理
n = 128;
match_point_index_set = ones(n,1)*nan;
proj_x_set = ones(n,1)*nan;
proj_y_set = ones(n,1)*nan;
proj_heading_set = ones(n,1)*nan;
proj_kappa_set = ones(n,1)*nan;

%两种情况：第一次遍历，非第一次遍历
%声明两个全局变量，第一个用来判断是否初次运行，第二个用来存储上次匹配点集合
persistent is_first_run
persistent pre_match_point_index_set
persistent pre_x_set
persistent pre_y_set
persistent pre_frenet_x_set;
persistent pre_frenet_y_set;
persistent pre_frenet_heading_set;

if isempty(is_first_run)
    is_first_run = 0;
    pre_match_point_index_set = ones(n,1)*nan;
    %遍历每一个点寻找匹配点
    start_search_index = 1;
    for i = 1:length(x_set)
        if isnan(x_set(i))
            break;
        end
        increase_count = 0;
        min_distant = inf;
        for j = start_search_index:length(frenet_x_set)
            distant = (x_set(i)-frenet_x_set(j))^2+(y_set(i)-frenet_y_set(j))^2;
            if distant < min_distant
                min_distant = distant;
                increase_count = 0;
                match_point_index_set(i) = j;
            else
                increase_count = increase_count+1;
            end
            %第一次遍历连续增加50次停止
            if increase_count > 50
                break;
            end
        end
        %通过匹配点计算投影点
        %计算匹配点的位矢及方向向量
        vector_match_point = [frenet_x_set(match_point_index_set(i));frenet_y_set(match_point_index_set(i))];
        vector_match_point_direction = [cos(frenet_heading_set(match_point_index_set(i)));sin(frenet_heading_set(match_point_index_set(i)))];
        vector_d = [x_set(i);y_set(i)]-vector_match_point;
        ds = vector_d'*vector_match_point_direction;
        vector_ds = ds*vector_match_point_direction;
        vector_proj_point = vector_match_point+vector_ds;
        %计算投影点的x,y,heading,kappa
        proj_x_set(i) = vector_proj_point(1);
        proj_y_set(i) = vector_proj_point(2);
        proj_heading_set(i) = frenet_heading_set(match_point_index_set(i))+frenet_kapppa_set(match_point_index_set(i))*ds;
        proj_kappa_set(i) = frenet_kapppa_set(match_point_index_set(i));
    end
    pre_match_point_index_set = match_point_index_set;
    pre_frenet_x_set = frenet_x_set;
    pre_frenet_y_set = frenet_y_set;
    pre_frenet_heading_set = frenet_heading_set;
    pre_x_set = x_set;
    pre_y_set = y_set;
else
    %如果不是第一次遍历
    for i = 1:length(x_set)

        if isnan(x_set(i))
            break;
        end
        %下面这行代码有严重问题，需要投影的不仅是自车，还有障碍物
        %而第一次运行时传感器可能监测不到障碍物，即算法会跳过is first run分支执行else分支
        %此时pre_match_point_index_set中除了自车都是nan，所以需要修复
        start_search_index = pre_match_point_index_set(i);
        increase_count_limit = 5;

        %下面是修复一个bug，pre_match_point_index(i)与x_set(i)不一定是同一个障碍物
        square_dis = (x_set(i)-pre_x_set(i))^2+(y_set(i)-pre_y_set(i))^2;
        if square_dis > 36
            start_search_index = nan;
        end

        if isnan(start_search_index)
            %从第一个点开始遍历，并需要遍历50次防止取到局部极小值
            increase_count_limit = 50;
            start_search_index = 1;
        end

        increase_count = 0;
        min_distant = inf;
        %判断遍历方向
        vector_pre_match_point = [pre_frenet_x_set(start_search_index);pre_frenet_y_set(start_search_index)];
        vector_pre_match_point_direction = [cos(pre_frenet_heading_set(start_search_index));sin(pre_frenet_heading_set(start_search_index))];
        flag = ([x_set(i);y_set(i)]-vector_pre_match_point)'*vector_pre_match_point_direction;
        

        %正向遍历
        if flag > 0.001
            for j = start_search_index:length(frenet_x_set)
                distant = (x_set(i)-frenet_x_set(j))^2+(y_set(i)-frenet_y_set(j))^2;
                if distant < min_distant
                    min_distant = distant;
                    increase_count = 0;
                    match_point_index_set(i) = j;
                else
                    increase_count = increase_count+1;
                end
                %连续增加5次停止
                if increase_count > increase_count_limit
                    break;
                end
            end
            % %通过匹配点计算投影点
            % %计算匹配点的位矢及方向向量
            % vector_match_point = [frenet_x_set(match_point_index_set(i));frenet_y_set(match_point_index_set(i))];
            % vector_match_point_direction = [cos(frenet_heading_set(match_point_index_set(i)));sin(frenet_heading_set(match_point_index_set(i)))];
            % vector_d = [x_set(i);y_set(i)]-vector_match_point;
            % ds = vector_d'*vector_match_point_direction;
            % vector_ds = ds*vector_match_point_direction;
            % vector_proj_point = vector_match_point+vector_ds;
            % %计算投影点的x,y,heading,kappa
            % proj_x_set(i) = vector_proj_point(1);
            % proj_y_set(i) = vector_proj_point(2);
            % proj_heading_set(i) = frenet_heading_set(match_point_index_set(i))+frenet_kapppa_set(match_point_index_set(i))*ds;
            % proj_kappa_set(i) = frenet_kapppa_set(match_point_index_set(i));
        elseif flag < -0.001
            %反向遍历
             for j = start_search_index:-1:1
                distant = (x_set(i)-frenet_x_set(j))^2+(y_set(i)-frenet_y_set(j))^2;
                if distant < min_distant
                    min_distant = distant;
                    increase_count = 0;
                    match_point_index_set(i) = j;
                else
                    increase_count = increase_count+1;
                end
                %连续增加5次停止
                if increase_count > increase_count_limit
                    break;
                end
            end
        else
            match_point_index_set(i) = start_search_index;
        end

        %通过匹配点计算投影点
        %计算匹配点的位矢及方向向量
        vector_match_point = [frenet_x_set(match_point_index_set(i));frenet_y_set(match_point_index_set(i))];
        vector_match_point_direction = [cos(frenet_heading_set(match_point_index_set(i)));sin(frenet_heading_set(match_point_index_set(i)))];
        vector_d = [x_set(i);y_set(i)]-vector_match_point;
        ds = vector_d'*vector_match_point_direction;
        vector_ds = ds*vector_match_point_direction;
        vector_proj_point = vector_match_point+vector_ds;
        %计算投影点的x,y,heading,kappa
        proj_x_set(i) = vector_proj_point(1);
        proj_y_set(i) = vector_proj_point(2);
        proj_heading_set(i) = frenet_heading_set(match_point_index_set(i))+frenet_kapppa_set(match_point_index_set(i))*ds;
        proj_kappa_set(i) = frenet_kapppa_set(match_point_index_set(i));

    end
    pre_match_point_index_set = match_point_index_set;
    pre_frenet_x_set = frenet_x_set;
    pre_frenet_y_set = frenet_y_set;
    pre_frenet_heading_set = frenet_heading_set;
    pre_x_set = x_set;
    pre_y_set = y_set;
end

== matlab function testemplanner_cs/Audi_A8_Sedan_1/decision&planning module1/EM Planner/path and speed merge ==
  data: s input; trajectory_x output; s_dot input; s_dot2 input; relative_time input; current_time input; path_s input; trajectory_x_init input; trajectory_y_init input; trajectory_heading_init input; trajectory_kappa_init input; trajectory_y output; trajectory_heading output; trajectory_kappa output; trajectory_speed output; trajectory_accel output; trajectory_time output
function [trajectory_x,trajectory_y,trajectory_heading,trajectory_kappa,trajectory_speed,trajectory_accel,trajectory_time] = ...
    fcn(s,s_dot,s_dot2,relative_time,current_time,path_s,trajectory_x_init,trajectory_y_init,trajectory_heading_init,trajectory_kappa_init)
% 该函数将合并path和speed
% 由于path 是 60个点，speed 有 401个点，合并后，path和speed有401个点，因此需要做插值
n = 401;
trajectory_x = zeros(n,1);
trajectory_y = zeros(n,1);
trajectory_heading = zeros(n,1);
trajectory_kappa = zeros(n,1);
trajectory_speed = zeros(n,1);

trajectory_accel = zeros(n,1);
index = 1;
% 由于trajectory_x_init中不是所有的值都有效，(有nan) 所以要找到有效值的范围
while ~isnan(trajectory_x_init(index)) 
    index = index + 1;
end
index = index - 1;
trajectory_time = zeros(n,1);
for i = 1:n-1
    %interp1 线性插值
    % 若 x = [1,2] y = [3,4]
    %interp1(x,y,1.5) 会得到3.5
    %interp1 的缺点是 在端点或超过端点的，结果为nan
    % interp1(x,y,2) 不会等于4 而是会等于nan
    % interp1(x,y,6) 也会等于nan，所以在端点处要单独处理
    trajectory_x(i) = interp1(path_s(1:index),trajectory_x_init(1:index),s(i));
    trajectory_y(i) = interp1(path_s(1:index),trajectory_y_init(1:index),s(i));
    trajectory_heading(i) = interp1(path_s(1:index),trajectory_heading_init(1:index),s(i));
    trajectory_kappa(i) = interp1(path_s(1:index),trajectory_kappa_init(1:index),s(i));
    trajectory_time(i) = relative_time(i) + current_time;%速度规划会得到相对时间，转换成绝对时间
    trajectory_speed(i) = s_dot(i);
    trajectory_accel(i) = s_dot2(i);
end
% 端点单独处理
trajectory_x(end) = trajectory_x_init(end);
trajectory_y(end) = trajectory_y_init(end);
trajectory_heading(end) = trajectory_heading_init(end);
trajectory_kappa(end) = trajectory_kappa_init(end);
trajectory_time(end) = relative_time(end) + current_time;
trajectory_speed(end) = s_dot(end);
trajectory_accel(end) = s_dot2(end);

== matlab function testemplanner_cs/Audi_A8_Sedan_1/decision&planning module1/EM Planner/plot1 ==
  data: dp_s input; dp_l input; qp_s input; qp_l input; l_min input; l_max input; obs_s_set input; obs_l_set input; start_s input; start_l input; start_dl input; centre_line input
function  fcn(dp_s,dp_l,qp_s,qp_l,l_min,l_max,obs_s_set,obs_l_set,start_s,start_l,start_dl, centre_line)
coder.extrinsic("plot","axis","figure","drawnow","cla","fill");

obs_length = 5;
obs_width = 2;
host_l = 6;
host_w = 1.63;
cla;
host_p1_l = start_l + sin(atan(start_dl)) * host_l /2 + host_w/2 * cos(atan(start_dl));
host_p1_s = start_s + cos(atan(start_dl)) * host_l /2 - host_w/2 * sin(atan(start_dl));
host_p2_l = start_l + sin(atan(start_dl)) * host_l /2 - host_w/2 * cos(atan(start_dl));
host_p2_s = start_s + cos(atan(start_dl)) * host_l /2 + host_w/2 * sin(atan(start_dl));
host_p3_l = start_l - sin(atan(start_dl)) * host_l /2 + host_w/2 * cos(atan(start_dl));
host_p3_s = start_s - cos(atan(start_dl)) * host_l /2 - host_w/2 * sin(atan(start_dl));
host_p4_l = start_l - sin(atan(start_dl)) * host_l /2 - host_w/2 * cos(atan(start_dl));
host_p4_s = start_s - cos(atan(start_dl)) * host_l /2 + host_w/2 * sin(atan(start_dl));
host_area_x = [host_p1_s;host_p2_s;host_p4_s;host_p3_s];
host_area_y = [host_p1_l;host_p2_l;host_p4_l;host_p3_l];
fill(host_area_x,host_area_y,[0 1 1]);
hold on
plot(dp_s,dp_l,'r');
plot(dp_s, centre_line, 'g');
plot(qp_s,qp_l,'b');
plot(dp_s,l_min,dp_s,l_max);
axis([-8 70 -10 10]);

for i = 1:length(obs_s_set)
    if isnan(obs_s_set(i))
        break;
    end
    obs_p1_s = obs_s_set(i) + obs_length/2;
    obs_p1_l = obs_l_set(i) + obs_width/2;
    obs_p2_s = obs_s_set(i) + obs_length/2;
    obs_p2_l = obs_l_set(i) - obs_width/2;
    obs_p3_s = obs_s_set(i) - obs_length/2;
    obs_p3_l = obs_l_set(i) + obs_width/2;
    obs_p4_s = obs_s_set(i) - obs_length/2;
    obs_p4_l = obs_l_set(i) - obs_width/2;
    obs_area_s = [obs_p1_s;obs_p2_s;obs_p4_s;obs_p3_s];
    obs_area_l = [obs_p1_l;obs_p2_l;obs_p4_l;obs_p3_l];
    fill(obs_area_s,obs_area_l,[0 0 0]);
end

== matlab function testemplanner_cs/Audi_A8_Sedan_1/decision&planning module1/EM Planner/simple speed qp planning ==
  data: plan_start_s_dot input; s_init output; plan_start_s_dot2 input; s_end input; recommend_T input; s_dot_init output; s_dot2_init output; relative_time_init output
function [s_init,s_dot_init,s_dot2_init,relative_time_init] = fcn(plan_start_s_dot,plan_start_s_dot2,s_end,recommend_T)
%简单速度二次规划
coder.extrinsic("quadprog")
n = 51;
s_init = zeros(n,1);
s_dot_init = zeros(n,1);
s_dot2_init = zeros(n,1);
relative_time_init = zeros(n,1);

Aeq = zeros(3*n,2*n - 2);
beq = zeros(2*n - 2,1);
lb = ones(3*n,1);
ub = lb;
dt = recommend_T/(n-1);
A_sub =[1,0;
        dt,1;
        (1/3)*dt^2,(1/2)*dt;
        -1,0;
        0,-1;
        (1/6)*dt^2,dt/2];
for i = 1:n - 1
    Aeq(3*i-2:3*i+3,2*i-1:2*i) = A_sub;
end

for i = 1:n
   lb(3*i - 2) = -inf;
   lb(3*i - 1) = 0;
   lb(3*i) = -8;
   ub(3*i - 2) = inf;
   ub(3*i - 1) = 50;
   ub(3*i) = 2;
end
lb(1) = 0;
lb(2) = plan_start_s_dot;
lb(3) = plan_start_s_dot2;
ub(1) = lb(1);
ub(2) = lb(2);
ub(3) = lb(3);
lb(3*n - 2) = s_end;
ub(3*n - 2) = s_end;
A3 = zeros(3*n,3*n);
A4 = zeros(3*n,n - 1);
A4_sub =[0;0;1;0;0;-1];
for i = 1:n - 1
   A3(3*i,3*i) = 1;
   A4(3*i-2:3*i+3,i:i) = A4_sub;
end
A3(3*n,3*n) = 1;
H = A3 + 100*(A4*A4');
H = 2*H;
f = zeros(3*n,1);
X = quadprog(H,f,[],[],Aeq',beq,lb,ub);
for i = 1:n
   s_init(i) = X(3*i - 2);
   s_dot_init(i) = X(3*i - 1);
   s_dot2_init(i) = X(3*i);
   relative_time_init(i) = (i - 1)*dt;
end

== matlab function testemplanner_cs/Audi_A8_Sedan_1/decision&planning module1/EM Planner/stitch trajectory ==
  data: trajectory_x input; trajectory_x_final output; trajectory_y input; trajectory_heading input; trajectory_kappa input; trajectory_speed input; trajectory_accel input; trajectory_time input; stitch_x input; stitch_y input; stitch_heading input; stitch_kappa input; stitch_speed input; stitch_accel input; stitch_time input; trajectory_y_final output; trajectory_heading_final output; trajectory_kappa_final output; trajectory_speed_final output; trajectory_accel_final output; trajectory_time_final output
function [trajectory_x_final,trajectory_y_final,trajectory_heading_final,trajectory_kappa_final,...
          trajectory_speed_final,trajectory_accel_final,trajectory_time_final] = fcn(trajectory_x,...
          trajectory_y,trajectory_heading,trajectory_kappa,trajectory_speed,trajectory_accel,trajectory_time,...
          stitch_x,stitch_y,stitch_heading,stitch_kappa,stitch_speed,stitch_accel,stitch_time)
% 轨迹拼接，把stitch trajectory 拼到规划完成的轨迹上
n = 401 + 20;
trajectory_x_final = zeros(n,1);
trajectory_y_final = zeros(n,1);
trajectory_heading_final = zeros(n,1);
trajectory_kappa_final = zeros(n,1);
trajectory_speed_final = zeros(n,1);
trajectory_accel_final = zeros(n,1);
trajectory_time_final = zeros(n,1);

trajectory_x_final = [stitch_x;trajectory_x];
trajectory_y_final = [stitch_y;trajectory_y];
trajectory_heading_final = [stitch_heading;trajectory_heading];
trajectory_kappa_final = [stitch_kappa;trajectory_kappa];
trajectory_speed_final = [stitch_speed;trajectory_speed];
trajectory_accel_final = [stitch_accel;trajectory_accel];
trajectory_time_final = [stitch_time;trajectory_time];
